simulink model "Wrapper_activation_condition_check"  (R2022b)
settings: Solver=FixedStepDiscrete  StartTime=0.0  StopTime=inf  FixedStep=0.2  RelTol=1e-3
settings Model: Tag=BTC_SUBSYSTEM_REF_WRAPPER  Creator=developer  LastModifiedBy=developer
settings SolverCC: AlgebraicLoopSolver=TrustRegion
settings OptimizationCC: BlockReduction=off  ConditionallyExecuteInputs=off  DefaultParameterBehavior=Inlined  EnhancedBackFolding=on  PassReuseOutputArgsAs=Individual arguments  ZeroExternalMemoryAtStartup=off  ZeroInternalMemoryAtStartup=off  OptimizeBlockOrder=speed  DifferentSizesBufferReuse=on  OptimizationCustomize=off  EfficientTunableParamExpr=on
settings DebuggingCC: ParameterTunabilityLossMsg=error  UnconnectedInputMsg=warning  UnconnectedOutputMsg=warning  UnconnectedLineMsg=warning  BusObjectLabelMismatch=error  StrictBusMsg=ErrorOnBusTreatedAsVector  NonBusSignalsTreatedAsBus=error  SFMachineParentedDataDiag=warning
settings SFSimCC: MATLABDynamicMemAlloc=off  CustomCodeUndefinedFunction=UseInterfaceOnly
settings RTWCC: Description=Embedded Coder  SystemTargetFile=ert.tlc  TemplateMakefile=ert_default_tmf
settings CodeAppCC: ForceParamTrailComments=on  IgnoreCustomStorageClasses=off  MaxIdLength=256  OperatorAnnotations=on  SimulinkDataObjDesc=on  SFDataObjDesc=on  CustomSymbolStrGlobalVar=w_$R$N$M  CustomSymbolStrType=w_$N$R$M_T  InsertBlockDesc=on
settings ERTTargetCC: TargetLangStandard=C99 (ISO)  GenerateSampleERTMain=on  InlinedParameterPlacement=NonHierarchical  ERTCustomFileTemplate=example_file_process.tlc

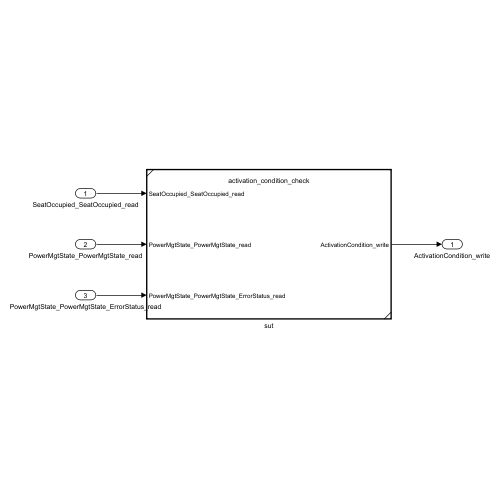
[thumbnail: Simulink's stored preview of the top-level diagram]
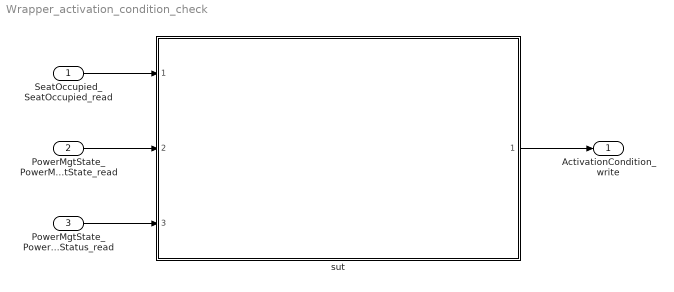
== system Wrapper_activation_condition_check ==
  SeatOccupied_SeatOccupied_read : Inport  OutDataTypeStr=boolean  PortDimensions=1
  PowerMgtState_PowerMgtState_read : Inport  Port=2  OutDataTypeStr=Enum:IDT_PowerState  PortDimensions=1
  PowerMgtState_PowerMgtState_ErrorStatus_read : Inport  Port=3  OutDataTypeStr=double  PortDimensions=1
  sut : Subsystem  TreatAsAtomicUnit=on  ReferencedSubsystem=activation_condition_check
  ActivationCondition_write : Outport  OutDataTypeStr=boolean  PortDimensions=1
  wires:
  SeatOccupied_SeatOccupied_read/1 -> sut/1
  PowerMgtState_PowerMgtState_read/1 -> sut/2
  PowerMgtState_PowerMgtState_ErrorStatus_read/1 -> sut/3
  sut/1 -> ActivationCondition_write/1
